simulink model "La1b_closed_multiple_graphs_ramp"  (R2024b)
settings: Solver=VariableStepAuto  StartTime=0.0  StopTime=40  RelTol=1e-3
values from neighbouring files (symbols this model uses):
  b = 666.1*10^-6    (= 0.0006661)    [Lab1b.m]
  J = 0.0081    [Lab1b.m]
  K_e = 0.094    [Lab1b.m]
  K_t = 0.094    [Lab1b.m]
  La = 528e-6    (= 0.000528)    [Lab1b.m]
  Ra = 0.649    [Lab1b.m]
libraries: simulink x1
settings Model: Creator=camer  LastModifiedBy=camer

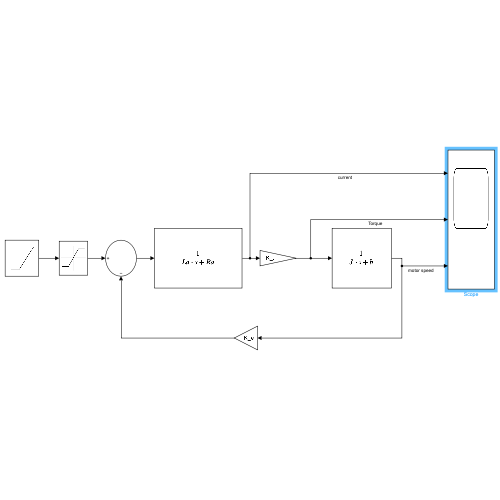
[thumbnail: Simulink's stored preview of the top-level diagram]
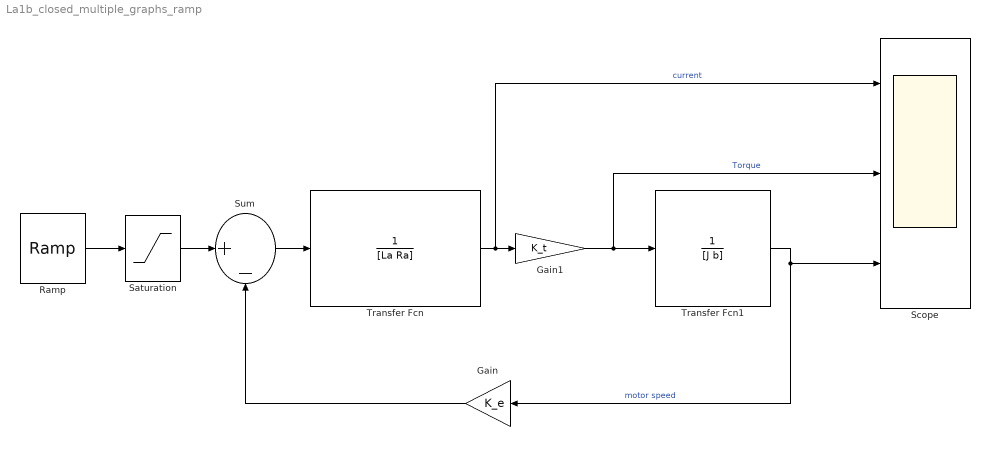
== system La1b_closed_multiple_graphs_ramp ==
  Gain : Gain  Gain=K_e
  Gain1 : Gain  Gain=K_t
  Ramp : simulink/Sources/Ramp  slope=4  start=2  InitialOutput=0
  Saturation : Saturate  UpperLimit=60
  Scope : Scope  NumInputPorts=3
  Sum : Sum  Inputs=|+-
  Transfer Fcn : TransferFcn  Denominator=[La Ra]
  Transfer Fcn1 : TransferFcn  Denominator=[J b]
  wires:
  Transfer Fcn1/1 -> Gain/1, Scope/3  "motor speed"
  Sum/1 -> Transfer Fcn/1
  Gain1/1 -> Scope/2, Transfer Fcn1/1  "Torque"
  Transfer Fcn/1 -> Scope/1, Gain1/1  "current"
  Gain/1 -> Sum/2
  Ramp/1 -> Saturation/1
  Saturation/1 -> Sum/1
